simulink model "Rot_Pen_PID"  (R2017a)
settings: Solver=VariableStepAuto  StartTime=0.0  StopTime=10.0  RelTol=1e-3
values from neighbouring files (symbols this model uses):
  A = [[0 , 0 , 1 , 0] ... (first row only)    [RotPen.m]
  B = [0 ; 0 ; Kt*(Jp+Mp*lp^2)/Rm/(Jeq*Jp+Jeq*Mp*lp^2+Mp*r^2*Jp) ; Mp*lp*Kt*r/Rm/(Jeq*Jp+Jeq*Mp*lp^2+Mp*r^2*Jp)]    [RotPen.m]
  C = [[1 0 0 0] ... (first row only)    [RotPen.m]
  D = [0 ; 0 ; 0 ; 0]    [RotPen.m]
  IC = [0 0.2 0 0]    [RotPen.m]
libraries: simulink x2
settings Model: Creator=Fouad  LastModifiedBy=Fouad

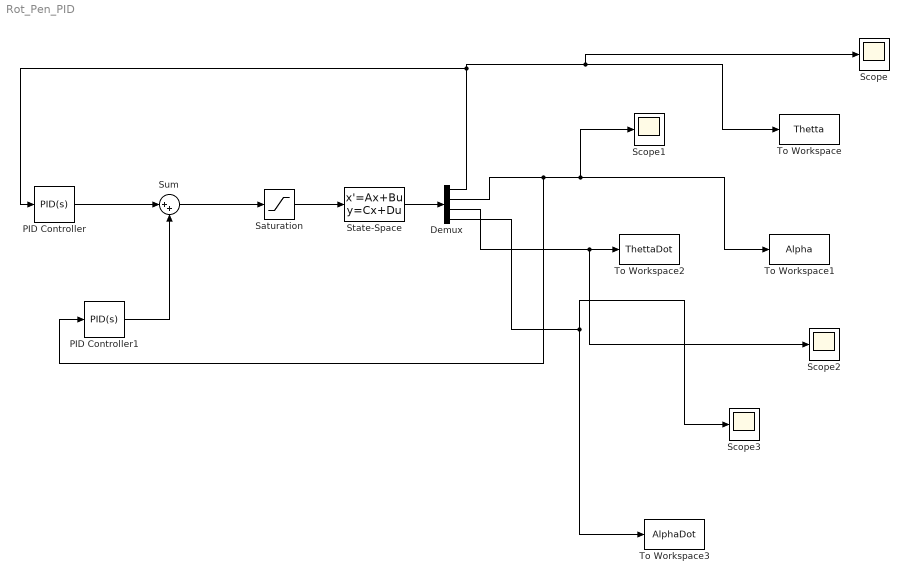
== system Rot_Pen_PID ==
  Demux : Demux
  PID Controller : simulink/Continuous/PID Controller  Controller=PID  TimeDomain=Continuous-time  SampleTime=-1  IntegratorMethod=Forward Euler  FilterMethod=Forward Euler  Form=Parallel  UseFilter=on  ControllerParametersSource=internal  P=0.00226459425342817  I=2.70054690835237e-07  D=4.06928976864629  N=0.0414866807129857  InitialConditionSource=internal  InitialConditionForIntegrator=0  InitialConditionForFilter=0  ExternalReset=none  LimitOutput=off  UpperSaturationLimit=inf  LowerSaturationLimit=-inf  LinearizeAsGain=on  AntiWindupMode=none  Kb=1  TrackingMode=off  Kt=1  PParamMin=[]  PParamMax=[]  IParamMin=[]  IParamMax=[]  DParamMin=[]  DParamMax=[]  NParamMin=[]  NParamMax=[]  KbParamMin=[]  KbParamMax=[]  KtParamMin=[]  KtParamMax=[]  POutMin=[]  POutMax=[]  IOutMin=[]  IOutMax=[]  DOutMin=[]  DOutMax=[]  NOutMin=[]  NOutMax=[]  KbOutMin=[]  KbOutMax=[]  KtOutMin=[]  KtOutMax=[]  IntegratorOutMin=[]  IntegratorOutMax=[]  FilterOutMin=[]  FilterOutMax=[]  SumOutMin=[]  SumOutMax=[]  SumI1OutMin=[]  SumI1OutMax=[]  SumI2OutMin=[]  SumI2OutMax=[]  SumI3OutMin=[]  SumI3OutMax=[]  SumDOutMin=[]  SumDOutMax=[]  SaturationOutMin=[]  SaturationOutMax=[]  IntegratorContinuousStateAttributes=''  IntegratorStateMustResolveToSignalObject=off  IntegratorRTWStateStorageClass=Auto  FilterContinuousStateAttributes=''  FilterStateMustResolveToSignalObject=off  FilterRTWStateStorageClass=Auto  DifferentiatorICPrevScaledInput=0  DifferentiatorOutMin=[]  DifferentiatorOutMax=[]  InitialConditionSetting=State (most efficient)
  PID Controller1 : simulink/Continuous/PID Controller  Controller=PID  TimeDomain=Continuous-time  SampleTime=-1  IntegratorMethod=Forward Euler  FilterMethod=Forward Euler  Form=Parallel  UseFilter=on  ControllerParametersSource=internal  P=-2118458.11238048  I=-41.326250198697  D=-14758415775.2329  N=0.0290267992226422  InitialConditionSource=internal  InitialConditionForIntegrator=0  InitialConditionForFilter=0  ExternalReset=none  LimitOutput=off  UpperSaturationLimit=inf  LowerSaturationLimit=-inf  LinearizeAsGain=on  AntiWindupMode=none  Kb=1  TrackingMode=off  Kt=1  PParamMin=[]  PParamMax=[]  IParamMin=[]  IParamMax=[]  DParamMin=[]  DParamMax=[]  NParamMin=[]  NParamMax=[]  KbParamMin=[]  KbParamMax=[]  KtParamMin=[]  KtParamMax=[]  POutMin=[]  POutMax=[]  IOutMin=[]  IOutMax=[]  DOutMin=[]  DOutMax=[]  NOutMin=[]  NOutMax=[]  KbOutMin=[]  KbOutMax=[]  KtOutMin=[]  KtOutMax=[]  IntegratorOutMin=[]  IntegratorOutMax=[]  FilterOutMin=[]  FilterOutMax=[]  SumOutMin=[]  SumOutMax=[]  SumI1OutMin=[]  SumI1OutMax=[]  SumI2OutMin=[]  SumI2OutMax=[]  SumI3OutMin=[]  SumI3OutMax=[]  SumDOutMin=[]  SumDOutMax=[]  SaturationOutMin=[]  SaturationOutMax=[]  IntegratorContinuousStateAttributes=''  IntegratorStateMustResolveToSignalObject=off  IntegratorRTWStateStorageClass=Auto  FilterContinuousStateAttributes=''  FilterStateMustResolveToSignalObject=off  FilterRTWStateStorageClass=Auto  DifferentiatorICPrevScaledInput=0  DifferentiatorOutMin=[]  DifferentiatorOutMax=[]  InitialConditionSetting=State (most efficient)
  Saturation : Saturate  UpperLimit=18  LowerLimit=-18
  Scope{,1..3} (4 alike) : Scope
  State-Space : StateSpace  A=A  B=B  C=C  D=D  X0=IC
  Sum : Sum  Inputs=|++
  To Workspace : ToWorkspace  VariableName=Thetta  SampleTime=0.01
  To Workspace1 : ToWorkspace  VariableName=Alpha  SampleTime=0.01
  To Workspace2 : ToWorkspace  VariableName=ThettaDot  SampleTime=0.01
  To Workspace3 : ToWorkspace  VariableName=AlphaDot  SampleTime=0.01
  wires:
  State-Space/1 -> Demux/1
  Demux/1 -> PID Controller/1, Scope/1, To Workspace/1
  Demux/2 -> PID Controller1/1, Scope1/1, To Workspace1/1
  Demux/3 -> Scope2/1, To Workspace2/1
  Demux/4 -> Scope3/1, To Workspace3/1
  Saturation/1 -> State-Space/1
  PID Controller/1 -> Sum/1
  PID Controller1/1 -> Sum/2
  Sum/1 -> Saturation/1
